simulink model "aero_dap3dof"  (R2023a)
settings: Solver=FixedStepAuto  StartTime=0  StopTime=ic.t_runtime  FixedStep=rcs.clockt  RelTol=1e-3  AbsTol=1e-6
PreLoadFcn:
  | evalc('run("DevelopingTheApolloLunarModuleDigitalAutopilotExample.mlx");');
undefined symbols (not defined in the file or in its folder): deg, ic, juliandate, mission, moon, rad, rcs, s
libraries: aerolibconvert2 x5, simulink_extras x2, vrlib x2, aerolibtransform2 x1, sharedtransform x1, aero_libdap x1, aero_librcs x1
CloseFcn:
  | h=findobj('type','figure','Name','aero_dap3dof');if ~isempty(h);close(h);end
Description:
  | Apollo Lunar Module Digital Autopilot
settings Model: RequirementInfo=9  ExtModeTrigMode=oneshot  Creator=The MathWorks, Inc.  LastModifiedBy=The MathWorks, Inc.
settings SolverCC: AutoScaleAbsTol=off  AlgebraicLoopSolver=TrustRegion  MaxZcPerStep=1
settings DataIOCC: SaveFormat=Array  ReturnWorkspaceOutputs=off  SignalLoggingName=logsOut
settings OptimizationCC: BlockReduction=off  ExpressionDepthLimit=2147483647  InitFltsAndDblsToZero=on
settings DebuggingCC: SaveWithParameterizedLinksMsg=none  SignalResolutionControl=TryResolveAllWithWarning  MultiTaskDSMMsg=warning  MultiTaskCondExecSysMsg=none  SigSpecEnsureSampleTimeMsg=none  FcnCallInpInsideContextMsg=warning  UnconnectedInputMsg=warning  UnconnectedOutputMsg=warning  UnconnectedLineMsg=warning  StateNameClashWarn=warning  SFUnexpectedBacktrackingDiag=warning  SFNoUnconditionalDefaultTransitionDiag=warning  SFExecutionAtInitializationDiag=none  ArithmeticOperatorsInVariantConditions=warning
settings HardwareCC: ProdBitPerPointer=32  ProdBitPerSizeT=32  ProdBitPerPtrDiffT=32  ProdLargestAtomicFloat=None  ProdIntDivRoundTo=Undefined  ProdEndianess=Unspecified  ProdWordSize=32  ProdHWDeviceType=Specified
settings ModelReferenceCC: EnableRefExpFcnMdlSchedulingChecks=on  PropagateSignalLabelsOutOfModel=off
settings SFSimCC: SimUseLocalCustomCode=off  SimParseCustomCode=off  CustomCodeUndefinedFunction=UseInterfaceOnly
settings RTWCC: RTWUseLocalCustomCode=off  DLArmComputeVersion=19.05
settings CodeAppCC: StateflowObjectComments=on
settings GRTTargetCC: TargetLangStandard=C89/C90 (ANSI)
settings ConfigComp: CovMetricSettings=d  CovSaveCumulativeToWorkspaceVar=on  CovSaveSingleToWorkspaceVar=on  CovExternalEMLEnable=off

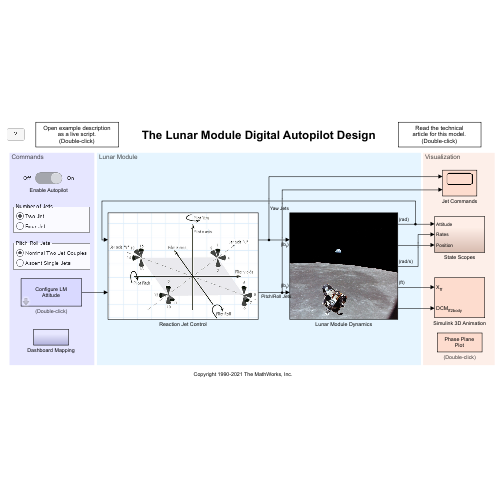
[thumbnail: Simulink's stored preview of the top-level diagram]
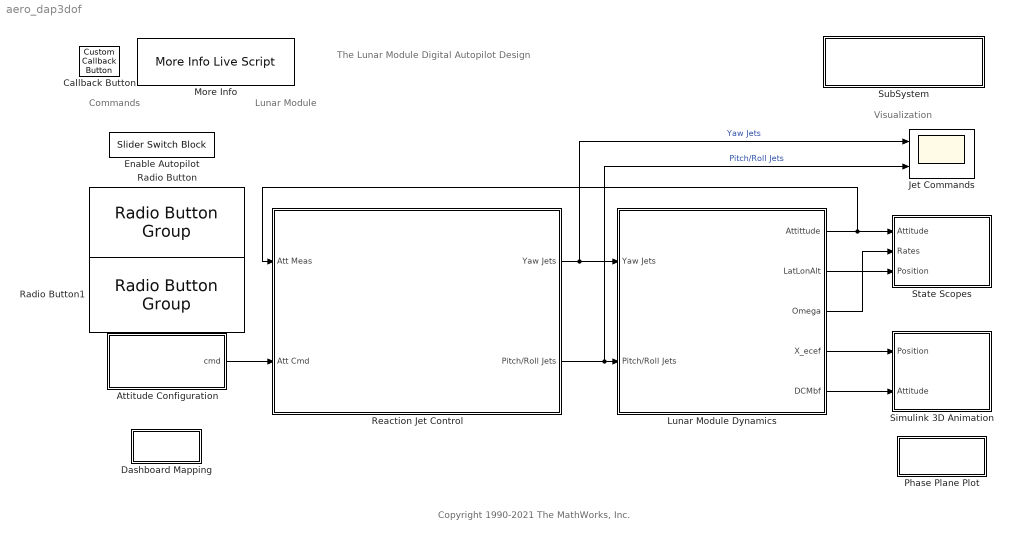
== system aero_dap3dof ==
  note: Lunar Module
  note: Visualization
  note: Commands
  note: The Lunar Module Digital Autopilot Design
  note: Copyright 1990-2021 The MathWorks, Inc.
  Attitude Configuration : Subsystem  mask(Configure LM Attitude){att_cmd=ic.euler_0 + [0 0 2], p_0=0.573, q_0=0.573, r_0=6.808}
      mask prompts: att_cmd "<html>Pilot commanded<br>attitude (roll, pitch, yaw)<br>[deg, deg, deg]</html>"; p_0 "Roll rate [deg/s]"; q_0 "Pitch rate [deg/s]"; r_0 "Yaw rate [deg/s]"
      settings: AttributesFormatString=(Double-click)
      mask Callback p_0:
      | pqr = [str2double(get_param(gcb, 'p_0')), ...
      |     str2double(get_param(gcb, 'q_0')),...
      |     str2double(get_param(gcb, 'r_0'))]';
      | 
      | evalin('base',['ic.pqr_0 = ' mat2str(pqr) ';']);
      mask Callback q_0:
      | pqr = [str2double(get_param(gcb, 'p_0')), ...
      |     str2double(get_param(gcb, 'q_0')),...
      |     str2double(get_param(gcb, 'r_0'))]';
      | 
      | evalin('base',['ic.pqr_0 = ' mat2str(pqr) ';']);
      mask Callback r_0:
      | pqr = [str2double(get_param(gcb, 'p_0')), ...
      |     str2double(get_param(gcb, 'q_0')),...
      |     str2double(get_param(gcb, 'r_0'))]';
      | 
      | evalin('base',['ic.pqr_0 = ' mat2str(pqr) ';']);
      mask DialogControl DescGroupVar1 Prompt: Pilot Commanded Body Attitude
      mask DialogControl DescTextVar_copy Prompt: Specify desired body attitude angles to send to digital autopilot.
      mask DialogControl ParameterGroupVar Prompt: Initial Body Angular Rates
      mask DialogControl DescTextVar Prompt: Vary the initial angular rates of the Lunar Module to investigate the response of the digital autopilot design.
      mask Display: disp('Configure LM\nAttitude')
  Callback Button : CustomCallbackButton  Configuration="{\"components\":[{\"name\":\"BackgroundImageComponent\",\"settings\":{\"image\":{\"size\":[0,0],\"src\":\"default\",\"srcOrientation\":\"Right\"},\"position\":[0,0,1,1]}},{\"name\":\"ButtonStateComponent\",\"settings\":{\"buttonType\":\"momentary\",\"clickFcn\":\"showExample('simulink_aerospace\\/DevelopingTheApolloLunarModuleDigitalAutopilotExample')\",\"onValue\":1,\"position\":[0,0,1,1],\"pressDelay\":\"500\",\"pressFcn\":\"\",\"repeatInterval\":\"0\",\"states\":[{\"horizontalAlignment\":\"center\",\"image\":{\"position\":[0,0,1,1],\"src\":\"default\",\"srcOrientation\":\"Right\"},\"label\":{\"color\":[0.01176470588,0.01176470588,0.01176470588,1],\"icon\":{\"size\":[0,0],\"src\":\"default\",\"srcOrientation\":\"Right\"},\"iconPlacement\":\"left\",\"text\":{\"content\":\"?\"}},\"labelOffset\":[0,0],\"verticalAlignment\":\"middle\"},{\"horizontalAlignment\":\"center\",\"image\":{\"position\":[0,0,1,1],\"src\":\"default\",\"srcOrientation\":\"Right\"},\"label\":{\"color\":[0.01176470588,0.01176470588,0.01176470588,1],\"icon\":{\"size\":[0,0],\"src\":\"default\",\"srcOrientation\":\"Right\"},\"iconPlacement\":\"left\",\"text\":{\"content\":\"?\"}},\"labelOffset\":[0,0],\"verticalAlignment\":\"middle\"},{\"horizontalAlignment\":\"center\",\"image\":{\"position\":[0,0,1,1],\"src\":\"default\",\"srcOrientation\":\"Right\"},\"label\":{\"color\":[0.01176470588,0.01176470588,0.01176470588,1],\"icon\":{\"size\":[0,0],\"src\":\"default\",\"srcOrientation\":\"Right\"},\"iconPlacement\":\"left\",\"text\":{\"content\":\"?\"}},\"labelOffset\":[0,0],\"verticalAlignment\":\"middle\"},{\"horizontalAlignment\":\"center\",\"image\":{\"position\":[0,0,1,1],\"src\":\"default\",\"srcOrientation\":\"Right\"},\"label\":{\"color\":[0.01176470588,0.01176470588,0.01176470588,1],\"icon\":{\"size\":[0,0],\"src\":\"default\",\"srcOrientation\":\"Right\"},\"iconPlacement\":\"left\",\"text\":{\"content\":\"?\"}},\"labelOffset\":[0,0],\"verticalAlignment\":\"middle\"}]}},{\"name\":\"ForegroundImageComponent\",\"settings\":{\"image\":{\"size\":[0,0],\"src\":\"default\",\"srcOrientation\":\"Right\"},\"isForeground\":1,\"position\":[0,0,1,1]}}],\"settings\":{\"BindingType\":\"standalone\",\"backgroundColor\":[244,244,244,1],\"backgroundOffset\":0.2,\"backgroundOpacity\":1,\"fixedAspectRatio\":\"off\",\"foregroundColor\":[0.01176470588,0.01176470588,0.01176470588,1],\"migratedFromLegacy\":true,\"useBackgroundColor\":true,\"variant\":\"callback\",\"version\":\"R2023a\"},\"type\":\"Button\"}"  CustomBackgroundColor="{\"color\":[0.9568627451,0.9568627451,0.9568627451],\"show\":true}"
  Dashboard Mapping : Subsystem
  Enable Autopilot : SliderSwitchBlock  LabelPosition=Hide
      settings: Values={{'Off', 'On'}, [0 1]}
  Jet Commands : Scope  NumInputPorts=2
  Lunar Module Dynamics : Subsystem
      mask Display: image('$imagefile'); % Use "Edit Image" on toolstrip to change.
  More Info : aero_libdap/More Info Live Script  SystemSampleTime=-1  VariantActivationTime=update diagram  Latency=0  AutoFrameSizeCalculation=off
  Phase Plane Plot : Subsystem  mask(Phase Plane Plot){enablePlot=on}
      mask prompts: enablePlot "Enable yaw phase plane plot"
      mask help: Enable yaw phase plane plotting during simulation.
      settings: AttributesFormatString=(Double-click)
      settings: OpenFcn=|
      | if ~builtin('license','test','virtual_reality_toolbox')
      |     set_param(gcb, 'enableVis', 'off');
      | end
      | open_system(gcb,'mask');
      mask Callback enablePlot:
      | if strcmp(get_param(gcb,'enablePlot'), 'on')
      |     set_param(gcb, 'Commented', 'off');
      | else
      |     set_param(gcb, 'Commented', 'on');
      | end
      mask Display: disp('Phase Plane\nPlot')
  Radio Button : RadioButtonGroup  LabelPosition=Hide  SelectedLabel=Two Jet  ButtonGroupName=Number of Jets
      settings: Values={{'Two Jet', 'Four Jet'}, [2 4]}
  Radio Button1 : RadioButtonGroup  LabelPosition=Hide  SelectedLabel=Nominal Two Jet Couples  ButtonGroupName=Pitch Roll Jets
      settings: Values={{'Nominal Two Jet Couples', 'Ascent Single Jets'}, [2 1]}
  Reaction Jet Control : Subsystem
      mask Display: image('$imagefile'); % Use "Edit Image" on toolstrip to change.
  Simulink 3D Animation : Subsystem  mask(Set Animation Properties){enableVis=on, visSampleTime=1}
      mask prompts: enableVis "Enable visualization with Simulink 3D Animation"; visSampleTime "Animation refresh rate:"
      mask help:
      | Change visualization properties used by Simulink 3D Animation. These settings are graphical only and do not affect simulation behavior.
      |
      | Hover over a dialog box for an explanation of the property.
      settings: OpenFcn=|
      | if ~builtin('license','test','virtual_reality_toolbox')
      |     set_param(gcb, 'enableVis', 'off');
      | end
      | open_system(gcb,'mask');
      mask Callback enableVis:
      | if strcmp(get_param(gcb,'enableVis'), 'on')
      |     enable = {'on', 'on'};
      |     set_param(gcb, 'Commented', 'off');
      | else
      |     enable = {'on', 'off'};
      |     set_param(gcb, 'Commented', 'on');
      | end
      | set_param(gcb,'MaskEnables', enable);
      | clear enable
      mask DialogControl vrOpenBtn Prompt: Open Simulink 3D Animation window
      mask DialogControl vrOpenBtn Callback: vrmfunc('FnOpen',getSimulinkBlockHandle([gcb '/VR Sink']));
      mask DialogControl visSampleTime Tooltip: <html>Sample time of animation window. Use this property to effectively speed up or slow down the animation. For example, a sample time of 1 causes the animation to update at every simulation time step. For a sample time of 20, the visualization will update every twentieth simulation time step. Maximum value is 1000.</html>
      mask Display:
      | port_label('input', 1, 'X_{ff}','texmode','on')
      | port_label('input', 2, 'DCM_{ff2body}','texmode','on')
  State Scopes : Subsystem
  SubSystem : Subsystem
      mask init:
      | dispstr = sprintf('Read the technical\narticle for this model.\n(Double-click)');
      settings: OpenFcn=web('https://www.mathworks.com/company/newsletters/articles/the-apollo-11-moon-landing-spacecraft-design-then-and-now.html')
      mask Display: disp(dispstr)
  wires:
  Lunar Module Dynamics/2(LatLonAlt) -> State Scopes/3(Position)
  Attitude Configuration/1(cmd) -> Reaction Jet Control/2(Att Cmd)
  Lunar Module Dynamics/1(Attittude) -> Reaction Jet Control/1(Att Meas), State Scopes/1(Attitude)
  Lunar Module Dynamics/3(Omega) -> State Scopes/2(Rates)
  Reaction Jet Control/2(Pitch/Roll Jets) -> Jet Commands/2, Lunar Module Dynamics/2(Pitch/Roll Jets)  "Pitch/Roll Jets"
  Reaction Jet Control/1(Yaw Jets) -> Jet Commands/1, Lunar Module Dynamics/1(Yaw Jets)  "Yaw Jets"
  Lunar Module Dynamics/4(X_ecef) -> Simulink 3D Animation/1(Position)
  Lunar Module Dynamics/5(DCMbf) -> Simulink 3D Animation/2(Attitude)

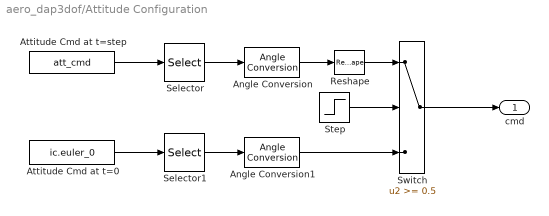
== system aero_dap3dof/Attitude Configuration ==
  Angle Conversion : aerolibconvert2/Angle Conversion  IU=deg  OU=rad
  Angle Conversion1 : aerolibconvert2/Angle Conversion  IU=deg  OU=rad
  Attitude Cmd at t=0 : Constant  Value=ic.euler_0  VectorParams1D=off
  Attitude Cmd at t=step : Constant  Value=att_cmd  VectorParams1D=off
  Reshape : Reshape
  Selector : Selector  InputPortWidth=3  IndexOptions=Index vector (dialog)  Indices=[3 1 2]  OutputSizes=1
  Selector1 : Selector  InputPortWidth=3  IndexOptions=Index vector (dialog)  Indices=[3 1 2]  OutputSizes=1
  Step : Step  Time=.25  SampleTime=0
  Switch : Switch  Threshold=0.5
  cmd : Outport  VectorParamsAs1DForOutWhenUnconnected=off
  wires:
  Reshape/1 -> Switch/1
  Angle Conversion/1 -> Reshape/1
  Step/1 -> Switch/2
  Attitude Cmd at t=0/1 -> Selector1/1
  Selector/1 -> Angle Conversion/1
  Switch/1 -> cmd/1
  Selector1/1 -> Angle Conversion1/1
  Angle Conversion1/1 -> Switch/3
  Attitude Cmd at t=step/1 -> Selector/1

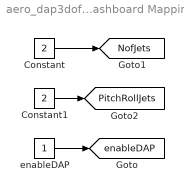
== system aero_dap3dof/Dashboard Mapping ==
  Constant : Constant  Value=2
  Constant1 : Constant  Value=2
  enableDAP : Constant
  tag scope: NofJets=global, PitchRollJets=global, enableDAP=global
  wires:
  Constant/1 -> [NofJets]
  Constant1/1 -> [PitchRollJets]
  enableDAP/1 -> [enableDAP]

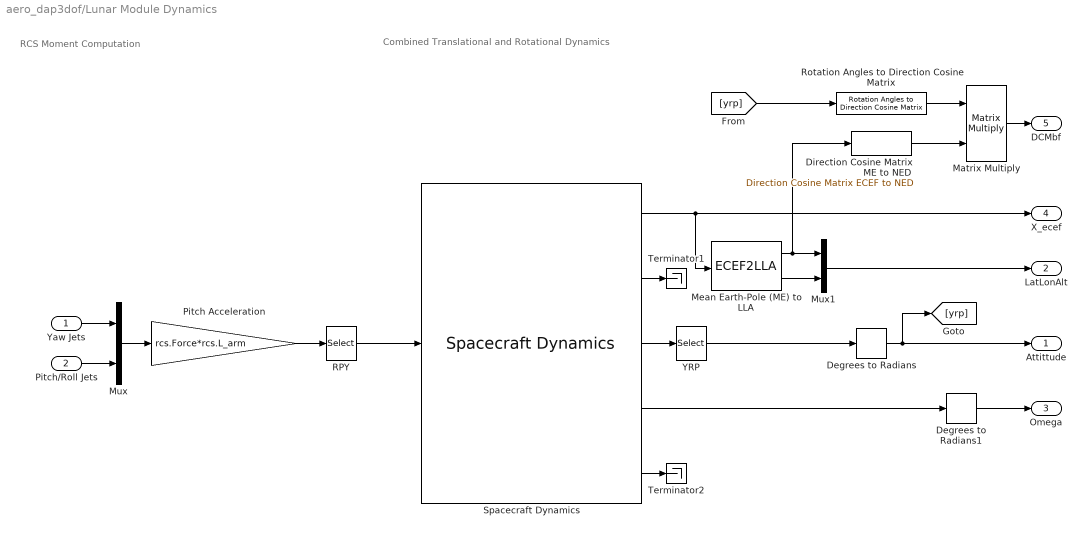
== system aero_dap3dof/Lunar Module Dynamics ==
  note: RCS Moment Computation
  note: Combined Translational and Rotational Dynamics
  Yaw Jets : Inport  Unit=lbf
  Pitch/Roll Jets : Inport  Port=2  Unit=lbf  PortDimensions=2
  Degrees to Radians : simulink_extras/Transformations/Degrees to Radians
  Degrees to Radians1 : simulink_extras/Transformations/Degrees to Radians
  Direction Cosine Matrix ME to NED : aerolibtransform2/Direction Cosine Matrix ECEF to NED
  Matrix Multiply : Product  Multiplication=Matrix(*)
  Mean Earth-Pole (ME) to LLA : ECEF2LLA  units=English  ptype=Custom  F=moon.f_moon  R=moon.r_moon_eq
  Mux : Mux  Inputs=2
  Mux1 : Mux  Inputs=2
  Pitch Acceleration : Gain  Gain=rcs.Force*rcs.L_arm  SaturateOnIntegerOverflow=on  OutDataTypeStr=Inherit: Same as input  ParamDataTypeStr=Inherit: Same as input
  RPY : Selector  InputPortWidth=3  IndexOptions=Index vector (dialog)  Indices=[2 3 1]  OutputSizes=1
  Rotation Angles to Direction Cosine Matrix : sharedtransform/Rotation Angles to Direction Cosine Matrix  rotationOrder=ZXY  aMode=aMode
  Spacecraft Dynamics : SpacecraftDynamics  forcesIn=off  outportFrame=Fixed-frame  startDate=juliandate(mission.t_descentInsertion)  mass=vehicle.mass_0  inertia=vehicle.inertia_0  stateFormatNum=ICRF state vector  inertialPosition=ic.pos_inertial  inertialVelocity=ic.vel_inertial  fixedPosition=[0 0 0]  fixedVelocity=[0 0 0]  attitudeFrame=NED  attitudeFormat=Euler angles  attitude=ic.euler_0  rotationOrder=XYZ  attitudeRate=ic.pqr_0  useGravGrad=off  centralBody=Moon  shDegree=60  units=English (ft/s)
      settings: AttributesFormatString=|
      | Central Body: %<centralBody>
      | Gravity Model: %<gravityModel> (%<moonSH>)
  Terminator1 : Terminator
  Terminator2 : Terminator
  YRP : Selector  InputPortWidth=3  IndexOptions=Index vector (dialog)  Indices=[3 1 2]  OutputSizes=1
  Attittude : Outport  Unit=rad  VectorParamsAs1DForOutWhenUnconnected=off
  LatLonAlt : Outport  Port=2  VectorParamsAs1DForOutWhenUnconnected=off
  Omega : Outport  Port=3  Unit=rad/s  VectorParamsAs1DForOutWhenUnconnected=off
  X_ecef : Outport  Port=4  Unit=ft  VectorParamsAs1DForOutWhenUnconnected=off
  DCMbf : Outport  Port=5  VectorParamsAs1DForOutWhenUnconnected=off
  wires:
  Spacecraft Dynamics/1 -> X_ecef/1, Mean Earth-Pole (ME) to LLA/1
  Mux/1 -> Pitch Acceleration/1
  Pitch Acceleration/1 -> RPY/1
  Direction Cosine Matrix ME to NED/1 -> Matrix Multiply/2
  Pitch/Roll Jets/1 -> Mux/2
  Mean Earth-Pole (ME) to LLA/2 -> Mux1/2
  Matrix Multiply/1 -> DCMbf/1
  Spacecraft Dynamics/4 -> Degrees to Radians1/1
  Degrees to Radians1/1 -> Omega/1
  [yrp] -> Rotation Angles to Direction Cosine Matrix/1
  Spacecraft Dynamics/5 -> Terminator2/1
  Rotation Angles to Direction Cosine Matrix/1 -> Matrix Multiply/1
  Spacecraft Dynamics/3 -> YRP/1
  YRP/1 -> Degrees to Radians/1
  Spacecraft Dynamics/2 -> Terminator1/1
  Degrees to Radians/1 -> [yrp], Attittude/1
  Yaw Jets/1 -> Mux/1
  Mean Earth-Pole (ME) to LLA/1 -> Mux1/1, Direction Cosine Matrix ME to NED/1
  Mux1/1 -> LatLonAlt/1
  RPY/1 -> Spacecraft Dynamics/1

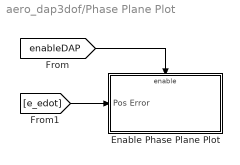
== system aero_dap3dof/Phase Plane Plot ==
  Enable Phase Plane Plot : Subsystem
  wires:
  [enableDAP] -> Enable Phase Plane Plot/Enable
  [e_edot] -> Enable Phase Plane Plot/1(Pos Error)

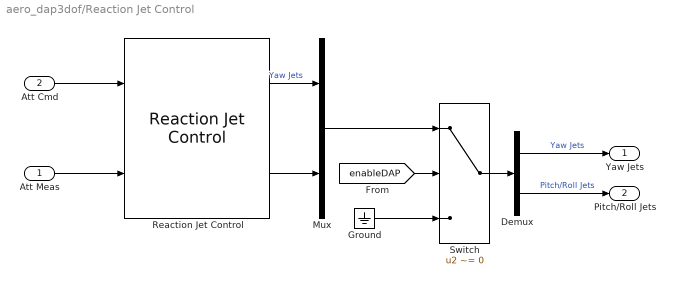
== system aero_dap3dof/Reaction Jet Control ==
  Att Meas : Inport
  Att Cmd : Inport  Port=2
  Demux : Demux  Outputs=[1 2]
  Ground : Ground
  Mux : Mux  Inputs=2
  Reaction Jet Control : aero_librcs/Reaction Jet Control  SystemSampleTime=-1  VariantActivationTime=update diagram  Latency=0  AutoFrameSizeCalculation=off
  Switch : Switch  Criteria=u2 ~= 0  SaturateOnIntegerOverflow=off  InputSameDT=off
  Yaw Jets : Outport  VectorParamsAs1DForOutWhenUnconnected=off
  Pitch/Roll Jets : Outport  Port=2  PortDimensions=2  VectorParamsAs1DForOutWhenUnconnected=off
  wires:
  Att Cmd/1 -> Reaction Jet Control/1
  Att Meas/1 -> Reaction Jet Control/2
  Demux/1 -> Yaw Jets/1  "Yaw Jets"
  Demux/2 -> Pitch/Roll Jets/1  "Pitch/Roll Jets"
  Ground/1 -> Switch/3
  Reaction Jet Control/1 -> Mux/1  "Yaw Jets"
  [enableDAP] -> Switch/2
  Mux/1 -> Switch/1
  Reaction Jet Control/2 -> Mux/2
  Switch/1 -> Demux/1

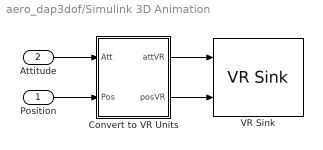
== system aero_dap3dof/Simulink 3D Animation ==
  Position : Inport
  Attitude : Inport  Port=2
  Convert to VR Units : Subsystem
  VR Sink : vrlib/VR Sink  InstantiateOnLoad=on  SampleTime=visSampleTime  ViewEnable=on  RemoteChange=off  RemoteView=off  FieldsWritten=LSAM.rotation.4.1.1.double#LSAM.translation.3.1.1.double  WorldFileName=Lander_Moon180_1.wrl  WorldDescription=Apollo Lunar Module Descent Animation  AutoView=on  VideoDimensions=[]  AllowVariableSize=off  FigureProperties="{'Position', 'Name', 'Viewpoint', 'CameraBound', 'CameraDirection', 'CameraPosition', 'CameraUpVector', 'ZoomFactor', 'Antialiasing', 'Headlight', 'Lighting', 'NavPanel', 'Sound', 'StatusBar', 'Stereo3D', 'Stereo3DCameraOffset', 'Stereo3DHIT', 'ToolBar', 'Textures', 'Transparency', 'Triad', 'Wireframe', 'NavZones', 'NavMode', 'NavSpeed', 'CaptureFileFormat', 'CaptureFileName', 'Record2DCompressMethod', 'Record2DCompressQuality', 'Record2D', 'Record2DFileName', 'Record2DFPS'; [4.3000000000000000e+01   1.2600000000000000e+02   5.7600000000000000e+02   3.5000000000000000e+02], 'Apollo Lunar Module Descent Animation', 'Follow Lander 1', 'on', [0.0000000000000000e+00   0.0000000000000000e+00  -1.0000000000000000e+00], [0.0000000000000000e+00   0.0000000000000000e+00   0.0000000000000000e+00], [0.0000000000000000e+00   1.0000000000000000e+00   0.0000000000000000e+00], [1.0000000000000000e+00], 'on', 'on', 'on', 'halfbar', 'on', 'on', 'off', [1.0000000149011612e-01], [0.0000000000000000e+00], 'on', 'on', 'on', 'none', 'off', 'off', 'examine', 'normal', 'tif', '%f_anim_%n.tif', 'auto', [7.5000000000000000e+01], 'off', '%f_anim_%n.avi', 'auto'}"
  wires:
  Attitude/1 -> Convert to VR Units/1(Att)
  Position/1 -> Convert to VR Units/2(Pos)
  Convert to VR Units/1(attVR) -> VR Sink/1
  Convert to VR Units/2(posVR) -> VR Sink/2

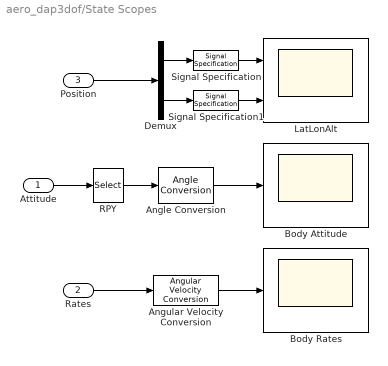
== system aero_dap3dof/State Scopes ==
  Attitude : Inport
  Rates : Inport  Port=2
  Position : Inport  Port=3
  Angle Conversion : aerolibconvert2/Angle Conversion  IU=rad  OU=deg
  Angular Velocity Conversion : aerolibconvert2/Angular Velocity Conversion  IU=rad/s  OU=deg/s
  Body Attitude : Scope
  Body Rates : Scope
  Demux : Demux  Outputs=[2 1]
  LatLonAlt : Scope  NumInputPorts=2
  RPY : Selector  InputPortWidth=3  IndexOptions=Index vector (dialog)  Indices=[2 3 1]  OutputSizes=1
  Signal Specification : SignalSpecification  Unit=deg
  Signal Specification1 : SignalSpecification  Unit=ft
  wires:
  Attitude/1 -> RPY/1
  Rates/1 -> Angular Velocity Conversion/1
  Demux/2 -> Signal Specification1/1
  Demux/1 -> Signal Specification/1
  Position/1 -> Demux/1
  Angle Conversion/1 -> Body Attitude/1
  Angular Velocity Conversion/1 -> Body Rates/1
  Signal Specification/1 -> LatLonAlt/1
  Signal Specification1/1 -> LatLonAlt/2
  RPY/1 -> Angle Conversion/1

== system aero_dap3dof/SubSystem ==

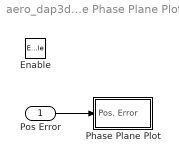
== system aero_dap3dof/Phase Plane Plot/Enable Phase Plane Plot ==
  Pos Error : Inport
  Enable : EnablePort  StatesWhenEnabling=reset
  Phase Plane Plot : Subsystem
  wires:
  Pos Error/1 -> Phase Plane Plot/1(Pos. Error)

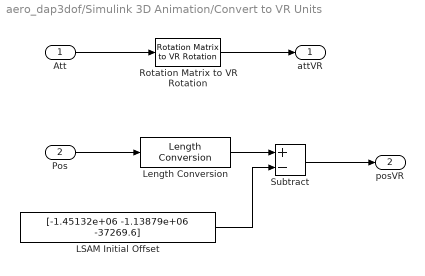
== system aero_dap3dof/Simulink 3D Animation/Convert to VR Units ==
  Att : Inport
  Pos : Inport  Port=2
  "LSAM Initial Offset " : Constant  Value=[-1.45132e+06 -1.13879e+06 -37269.6]
  Length Conversion : aerolibconvert2/Length Conversion  IU=ft  OU=m
  Rotation Matrix to VR Rotation : vrlib/Utilities/Rotation Matrix to VR Rotation  maxzero=1e-12
  Subtract : Sum  Inputs=+-
  attVR : Outport  VectorParamsAs1DForOutWhenUnconnected=off
  posVR : Outport  Port=2  VectorParamsAs1DForOutWhenUnconnected=off
  wires:
  Att/1 -> Rotation Matrix to VR Rotation/1
  Rotation Matrix to VR Rotation/1 -> attVR/1
  Pos/1 -> Length Conversion/1
  Length Conversion/1 -> Subtract/1
  Subtract/1 -> posVR/1
  "LSAM Initial Offset "/1 -> Subtract/2

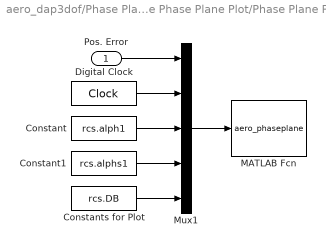
== system aero_dap3dof/Phase Plane Plot/Enable Phase Plane Plot/Phase Plane Plot ==
  Pos. Error : Inport
  Constant : Constant  Value=rcs.alph1
  Constant1 : Constant  Value=rcs.alphs1
  Constants for Plot : Constant  Value=rcs.DB
  Digital Clock : DigitalClock  SampleTime=rcs.delt
  MATLAB Fcn : MATLABFcn  MATLABFcn=aero_phaseplane  OutputDimensions=0
  Mux1 : Mux  Inputs=5
  wires:
  Mux1/1 -> MATLAB Fcn/1
  Pos. Error/1 -> Mux1/1
  Digital Clock/1 -> Mux1/2
  Constants for Plot/1 -> Mux1/5
  Constant/1 -> Mux1/3
  Constant1/1 -> Mux1/4
